simulink model "mavsim_chap13_gimbal_model"  (Simulink 8.8)
settings: Solver=ode45  StartTime=0.0  StopTime=400  RelTol=1e-3  EnableMultiTasking=on
InitFcn:
  | param_chap13
undefined symbols (not defined in the file or in its folder): camera, drawEnvironmentCamera, P, path_follow, path_manager, path_planner, point_gimbal
settings Model: SuppressorTable=22 serialization::archive 11 0 3 0 0 0 11 0  Creator=beard  LastModifiedBy=nmd89
settings OptimizationCC: ExpressionDepthLimit=2147483647  InitFltsAndDblsToZero=on
settings DebuggingCC: SolverPrmCheckMsg=warning
settings SFSimCC: SimParseCustomCode=off

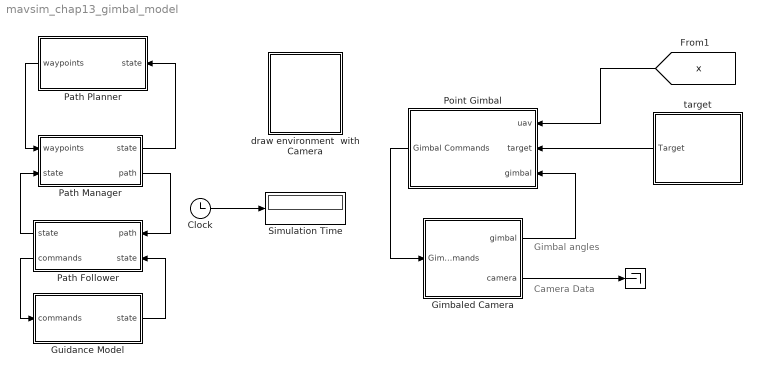
== system mavsim_chap13_gimbal_model ==
  note: Gimbal angles
  note: Camera Data
  " " : Terminator
  Clock : Clock
  Gimbaled Camera : Subsystem
      mask Display: image(imread('gimbal.jpg'))
  Guidance Model : Subsystem
  Path Follower : Subsystem
  Path Manager : Subsystem
  Path Planner : Subsystem
  Point Gimbal : Subsystem
  Simulation Time : Display
  draw environment  with Camera : Subsystem  mask{map=P.map, R_min=P.R_min, cam_fov=P.cam_fov}
      mask prompts: cam_fov "FOV of Camera"
      mask init:
      | % parameters for drawing aircraft
      |   % scale size
      |   size = 1;
      |   fuse_l1    = 7;
      |   fuse_l2    = 4;
      |   fuse_l3    = 15;
      |   fuse_w     = 2;
      |   wing_l     = 6;
      |   wing_w     = 20;
      |   tail_l     = 3;
      |   tail_h     = 3;
      |   tailwing_w = 10;
      |   tailwing_l = 3;
      |   % colors
      |   red     = [1, 0, 0];
      |   green   = [0, 1, 0];
      |   blue    = [0, 0, 1];
      |   yellow  = [1,1,0];
      |   magenta = [0, 1, 1];
      |   
      | 
      | % define vertices and faces for aircraft
      |   V = [...
      |     fuse_l1,             0,             0;...        % point 1
      |     fuse_l2,            -fuse_w/2,     -fuse_w/2;... % point 2     
      |     fuse_l2,             fuse_w/2,     -fuse_w/2;... % point 3     
      |     fuse_l2,             fuse_w/2,      fuse_w/2;... % point 4
      |     fuse_l2,            -fuse_w/2,      fuse_w/2;... % point 5
      |    -fuse_l3,             0,             0;...        % point 6
      |     0,                   wing_w/2,      0;...        % point 7
      |    -wing_l,              wing_w/2,      0;...        % point 8
      |    -wing_l,             -wing_w/2,      0;...        % point 9
      |     0,                  -wing_w/2,      0;...        % point 10
      |    -fuse_l3+tailwing_l,  tailwing_w/2,  0;...        % point 11
      |    -fuse_l3,             tailwing_w/2,  0;...        % point 12
      |    -fuse_l3,            -tailwing_w/2,  0;...        % point 13
      |    -fuse_l3+tailwing_l, -tailwing_w/2,  0;...        % point 14
      |    -fuse_l3+tailwing_l,  0,             0;...        % point 15
      |    -fuse_l3+tailwing_l,  0,             -tail_h;...  % point 16
      |    -fuse_l3,             0,             -tail_h;...  % point 17
      |   ];
      |   
      |   F = [...
      |         1,  2,  3,  1;... % nose-top
      |         1,  3,  4,  1;... % nose-left
      |         1,  4,  5,  1;... % nose-bottom
      |         1,  5,  2,  1;... % nose-right
      |         2,  3,  6,  2;... % fuselage-top
      |         3,  6,  4,  3;... % fuselage-left
      |         4,  6,  5,  4;... % fuselage-bottom
      |         2,  5,  6,  2;... % fuselage-right
      |         7,  8,  9, 10;... % wing
      |        11, 12, 13, 14;... % tailwing
      |         6, 15, 17, 17;... % tail
      |         
      |   ];  
      |   
      |   colors = [...
      |         yellow;... % nose-top
      |         yellow;... % nose-left
      |         yellow;... % nose-bottom
      |         yellow;... % nose-right
      |         blue;... % fuselage-top
      |         blue;... % fuselage-left
      |         red;... % fuselage-bottom
      |         blue;... % fuselage-right
      |         green;... % wing
      |         green;... % tailwing
      |         blue;... % tail
      |     ];
      | 
      |   V = size*V;   % rescale vertices
      mask Display: image(imread('tv.jpg'))
  target : Subsystem
      mask Display: image(imread('monstertruck.jpg'))
  wires:
  Clock/1 -> Simulation Time/1
  Path Follower/2(commands) -> Guidance Model/1(commands)
  Guidance Model/1(state) -> Path Follower/2(state)
  Path Manager/2(path) -> Path Follower/1(path)
  Path Follower/1("state ") -> Path Manager/2(state)
  Path Planner/1(waypoints) -> Path Manager/1(waypoints)
  Path Manager/1("state ") -> Path Planner/1(state)
  Point Gimbal/1(Gimbal Commands) -> Gimbaled Camera/1(Gimbal Commands)
  Gimbaled Camera/1(gimbal) -> Point Gimbal/3(gimbal)
  target/1(Target) -> Point Gimbal/2(target)
  Gimbaled Camera/2(camera) -> " "/1
  [x] -> Point Gimbal/1(uav)

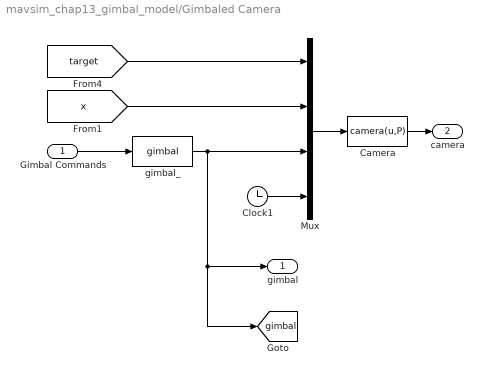
== system mavsim_chap13_gimbal_model/Gimbaled Camera ==
  Gimbal Commands : Inport
  Camera : MATLABFcn  MATLABFcn=camera(u,P)  OutputDimensions=3  SampleTime=1/P.cam_fps
  Clock1 : Clock
  Mux : Mux
  gimbal_ : S-Function  FunctionName=gimbal  Parameters=P  SFunctionDeploymentMode=off  EnableBusSupport=off
  gimbal : Outport
  camera : Outport  Port=2
  tag scope: gimbal=global
  wires:
  Mux/1 -> Camera/1
  [x] -> Mux/2
  Camera/1 -> camera/1
  [target] -> Mux/1
  Clock1/1 -> Mux/4
  Gimbal Commands/1 -> gimbal_/1
  gimbal_/1 -> Mux/3, gimbal/1, [gimbal]

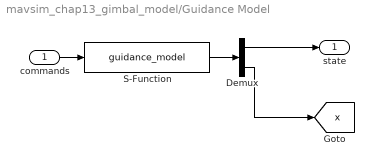
== system mavsim_chap13_gimbal_model/Guidance Model ==
  commands : Inport
  Demux : Demux  Outputs=[16;12]
  S-Function : S-Function  FunctionName=guidance_model  Parameters=P  SFunctionDeploymentMode=off  EnableBusSupport=off
  state : Outport
  tag scope: x=global
  wires:
  commands/1 -> S-Function/1
  S-Function/1 -> Demux/1
  Demux/1 -> state/1
  Demux/2 -> [x]

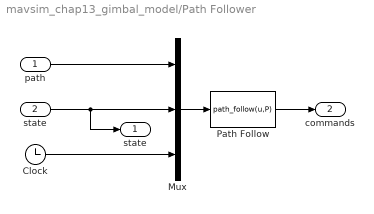
== system mavsim_chap13_gimbal_model/Path Follower ==
  path : Inport
  state : Inport  Port=2
  Clock : Clock
  Mux : Mux  Inputs=3
  Path Follow : MATLABFcn  MATLABFcn=path_follow(u,P)  OutputDimensions=4  SampleTime=P.Ts
  "state " : Outport
  commands : Outport  Port=2
  wires:
  Path Follow/1 -> commands/1
  Mux/1 -> Path Follow/1
  path/1 -> Mux/1
  Clock/1 -> Mux/3
  state/1 -> Mux/2, "state "/1

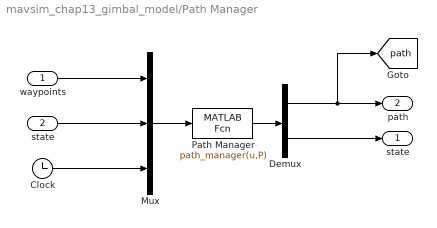
== system mavsim_chap13_gimbal_model/Path Manager ==
  waypoints : Inport
  state : Inport  Port=2
  Clock : Clock
  Demux : Demux  Outputs=[13;17]
  Mux : Mux  Inputs=3
  Path Manager : MATLABFcn  MATLABFcn=path_manager(u,P)  OutputDimensions=30  SampleTime=P.Ts
  "state " : Outport
  path : Outport  Port=2
  tag scope: path=global
  wires:
  Demux/2 -> "state "/1
  Demux/1 -> [path], path/1
  Path Manager/1 -> Demux/1
  waypoints/1 -> Mux/1
  state/1 -> Mux/2
  Clock/1 -> Mux/3
  Mux/1 -> Path Manager/1

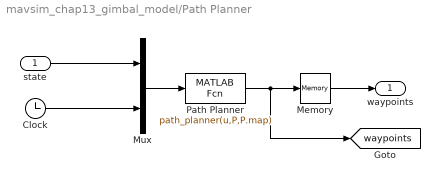
== system mavsim_chap13_gimbal_model/Path Planner ==
  state : Inport
  Clock : Clock
  Memory : Memory
  Mux : Mux  Inputs=2
  Path Planner : MATLABFcn  MATLABFcn=path_planner(u,P,P.map)  OutputDimensions=1+5*P.size_waypoint_array  SampleTime=100*P.Ts
  waypoints : Outport
  tag scope: waypoints=global
  wires:
  Mux/1 -> Path Planner/1
  Clock/1 -> Mux/2
  state/1 -> Mux/1
  Path Planner/1 -> Memory/1, [waypoints]
  Memory/1 -> waypoints/1

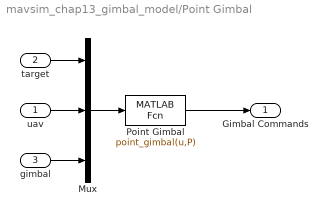
== system mavsim_chap13_gimbal_model/Point Gimbal ==
  uav : Inport
  target : Inport  Port=2
  gimbal : Inport  Port=3
  Mux : Mux  Inputs=3
  Point Gimbal : MATLABFcn  MATLABFcn=point_gimbal(u,P)  OutputDimensions=2  SampleTime=P.Ts
  Gimbal Commands : Outport
  wires:
  Mux/1 -> Point Gimbal/1
  uav/1 -> Mux/2
  Point Gimbal/1 -> Gimbal Commands/1
  target/1 -> Mux/1
  gimbal/1 -> Mux/3

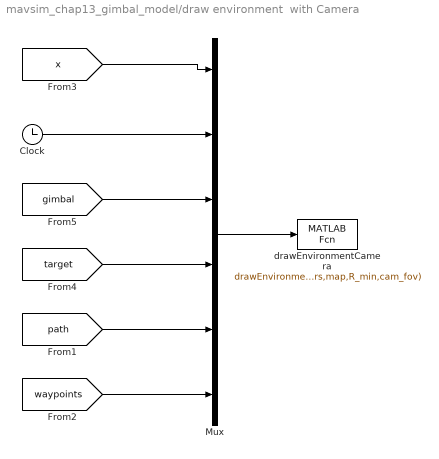
== system mavsim_chap13_gimbal_model/draw environment  with Camera ==
  Clock : Clock
  Mux : Mux  Inputs=6
  drawEnvironmentCamera : MATLABFcn  MATLABFcn=drawEnvironmentCamera(u,V,F,colors,map,R_min,cam_fov)  OutputDimensions=0  SampleTime=0.1
  wires:
  [target] -> Mux/4
  [gimbal] -> Mux/3
  [waypoints] -> Mux/6
  [path] -> Mux/5
  Mux/1 -> drawEnvironmentCamera/1
  [x] -> Mux/1
  Clock/1 -> Mux/2

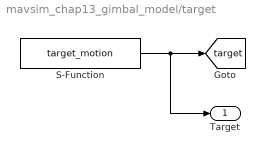
== system mavsim_chap13_gimbal_model/target ==
  S-Function : S-Function  FunctionName=target_motion  Parameters=P,P.map  SFunctionDeploymentMode=off  EnableBusSupport=off
  Target : Outport
  tag scope: target=global
  wires:
  S-Function/1 -> [target], Target/1
